simulink model "lead_car_stationary_ego_speedup25a"  (R2025a)
settings: Solver=VariableStepAuto  StartTime=0.0  StopTime=10.0  RelTol=1e-3
settings Model: Creator=jdcjd  LastModifiedBy=jdcjd

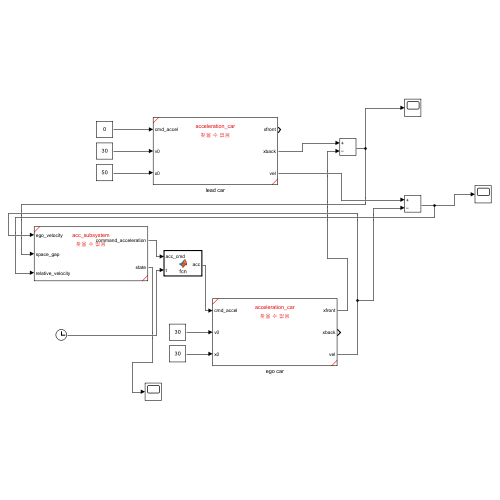
[thumbnail: Simulink's stored preview of the top-level diagram]
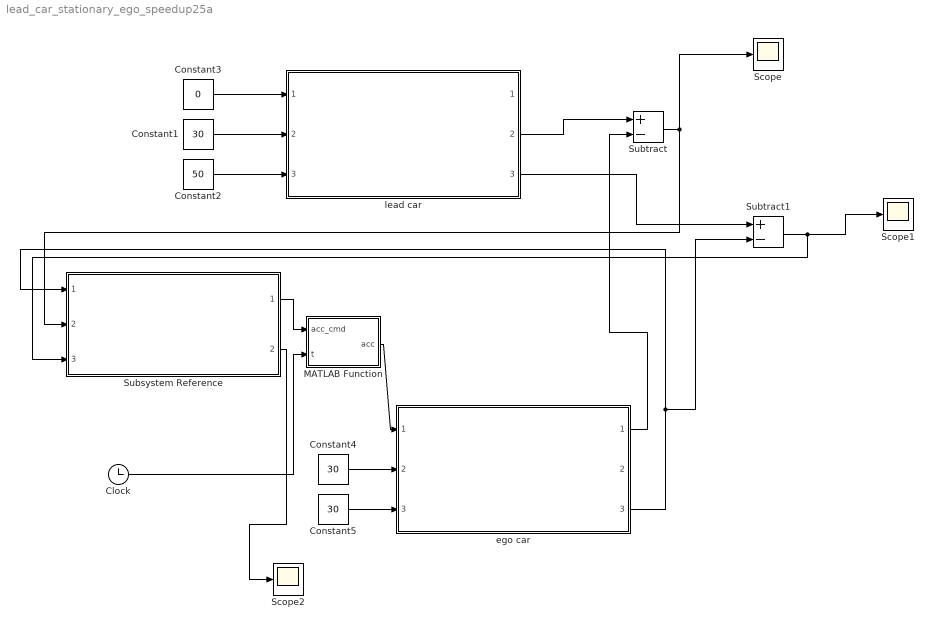
== system lead_car_stationary_ego_speedup25a ==
  Clock : Clock
  Constant1 : Constant  Value=30
  Constant2 : Constant  Value=50
  Constant3 : Constant  Value=0
  Constant4 : Constant  Value=30
  Constant5 : Constant  Value=30
  MATLAB Function : MATLAB Function  TreatAsAtomicUnit=on
  Scope : Scope
  Scope1 : Scope
  Scope2 : Scope
      settings: DataLoggingVariableName=ScopeData2
  Subsystem Reference : Subsystem  ReferencedSubsystem=acc_subsystem
  Subtract : Sum  Inputs=+-
  Subtract1 : Sum  Inputs=+-
  ego car : Subsystem  ReferencedSubsystem=acceleration_car
  lead car : Subsystem  ReferencedSubsystem=acceleration_car
  wires:
  Constant3/1 -> lead car/1
  Constant1/1 -> lead car/2
  Constant2/1 -> lead car/3
  lead car/3 -> Subtract1/1
  ego car/3 -> Subsystem Reference/1, Subtract1/2
  lead car/2 -> Subtract/1
  ego car/1 -> Subtract/2
  Subtract/1 -> Subsystem Reference/2, Scope/1
  Subtract1/1 -> Scope1/1, Subsystem Reference/3
  Constant5/1 -> ego car/3
  Constant4/1 -> ego car/2
  MATLAB Function/1(acc) -> ego car/1
  Subsystem Reference/1 -> MATLAB Function/1(acc_cmd)
  Clock/1 -> MATLAB Function/2(t)
  Subsystem Reference/2 -> Scope2/1

== matlab function lead_car_stationary_ego_speedup25a/MATLAB Function ==
  data: acc_cmd input; acc output; t input
function acc = fcn(acc_cmd, t)

acc = acc_cmd * t * 0.5;
end
